simulink model "Sistema_Mecanico_Simulink"  (R2025b)
settings: Solver=VariableStepAuto  StartTime=0.0  StopTime=20.0  RelTol=1e-3
settings Model: Creator=nachi  LastModifiedBy=nachi

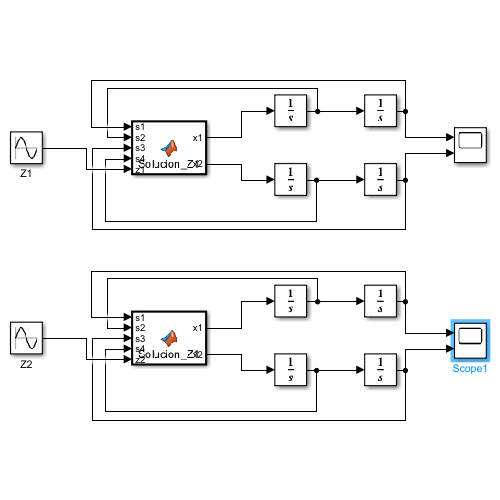
[thumbnail: Simulink's stored preview of the top-level diagram]
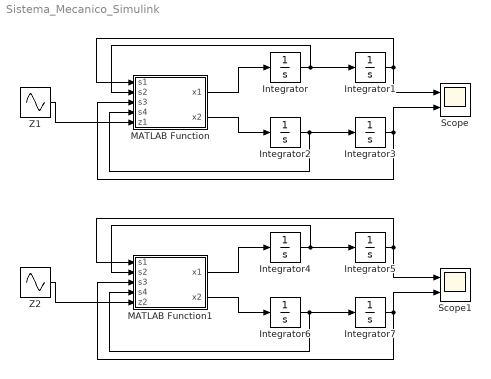
== system Sistema_Mecanico_Simulink ==
  Integrator{,1..7} (8 alike) : Integrator
  MATLAB Function : MATLAB Function  TreatAsAtomicUnit=on
  MATLAB Function1 : MATLAB Function  TreatAsAtomicUnit=on
  Scope : Scope  NumInputPorts=2
      settings: ActiveDisplayYMinimum=-0.219294312203999  ActiveDisplayYMaximum=0.18085573063456806
  Scope1 : Scope  NumInputPorts=2
      settings: ActiveDisplayYMinimum=-0.008076925877925939  ActiveDisplayYMaximum=0.033633448945054226
  Z1 : Sin  Amplitude=0.05  Frequency=0.5*pi  SampleTime=0
  Z2 : Sin  Amplitude=0.05  Frequency=20*pi  SampleTime=0
  wires:
  Integrator/1 -> MATLAB Function/2(s2), Integrator1/1
  Integrator2/1 -> MATLAB Function/4(s4), Integrator3/1
  Integrator1/1 -> Scope/1, MATLAB Function/1(s1)
  Integrator3/1 -> Scope/2, MATLAB Function/3(s3)
  MATLAB Function/1(x1) -> Integrator/1
  MATLAB Function/2(x2) -> Integrator2/1
  Z1/1 -> MATLAB Function/5(z1)
  Integrator6/1 -> MATLAB Function1/4(s4), Integrator7/1
  Integrator4/1 -> MATLAB Function1/2(s2), Integrator5/1
  Z2/1 -> MATLAB Function1/5(z2)
  MATLAB Function1/2(x2) -> Integrator6/1
  Integrator7/1 -> Scope1/2, MATLAB Function1/3(s3)
  Integrator5/1 -> Scope1/1, MATLAB Function1/1(s1)
  MATLAB Function1/1(x1) -> Integrator4/1

== matlab function Sistema_Mecanico_Simulink/MATLAB Function1 ==
  data: x1 output; s1 input; x2 output; s2 input; s3 input; s4 input; z2 input
function [x1, x2]= Solucion_Z2(s1, s2, s3, s4, z2)

    m1 = 290; b1 = 1000; m2 = 59; k1 = 16182;
    f = 0; k2 = 19000;

    x1 = - b1*s2/m1 ...
         + b1*s4/m1 ...
         - k1*s1/m1 ...
         + k1*s3/m1 ...
         + f/m1;

    x2 =   b1*s2/m2 ...
         - b1*s4/m2 ...
         + k1*s1/m2 ...
         - k1*s3/m2 ...
         - k2*s3/m2 ...
         - f/m2 ...
         + k2*z2/m2;

end

== matlab function Sistema_Mecanico_Simulink/MATLAB Function ==
  data: x1 output; s1 input; x2 output; s2 input; s3 input; s4 input; z1 input
function [x1, x2]= Solucion_Z1(s1, s2, s3, s4, z1)

    m1 = 290; b1 = 1000; m2 = 59; k1 = 16182;
    f = 0; k2 = 19000;

    x1 = - b1*s2/m1 ...
         + b1*s4/m1 ...
         - k1*s1/m1 ...
         + k1*s3/m1 ...
         + f/m1;

    x2 =   b1*s2/m2 ...
         - b1*s4/m2 ...
         + k1*s1/m2 ...
         - k1*s3/m2 ...
         - k2*s3/m2 ...
         - f/m2 ...
         + k2*z1/m2;

end
